simulink model "JUB27_MA"  (R2020b)
settings: Solver=FixedStepDiscrete  StartTime=0.0  StopTime=2*3600  FixedStep=Ts  RelTol=1e-3
values from neighbouring files (symbols this model uses):
  FreqAlvoIni = 55    [CarregaDados.m]
  NumCasasDecimais = 1    [CarregaDados.m]
  PMonAlvoIni = LimitaFaixa(PMonAlvoIni,FaixaPChegada)    [CarregaDados.m]
  Rede_Processo = load('weightsESNx_TR300_TVaz0.8_RaioE0.1.mat')    [CarregaDados.m]
  SNR = 40    [CarregaDados.m]
  Ts = 10    [CarregaDados.m]
undefined symbols (not defined in the file or in its folder): awgn, BTP, TabelaIsometricas, TabSimulador, UIni, YIni
settings Model: Creator=leize  LastModifiedBy=leize

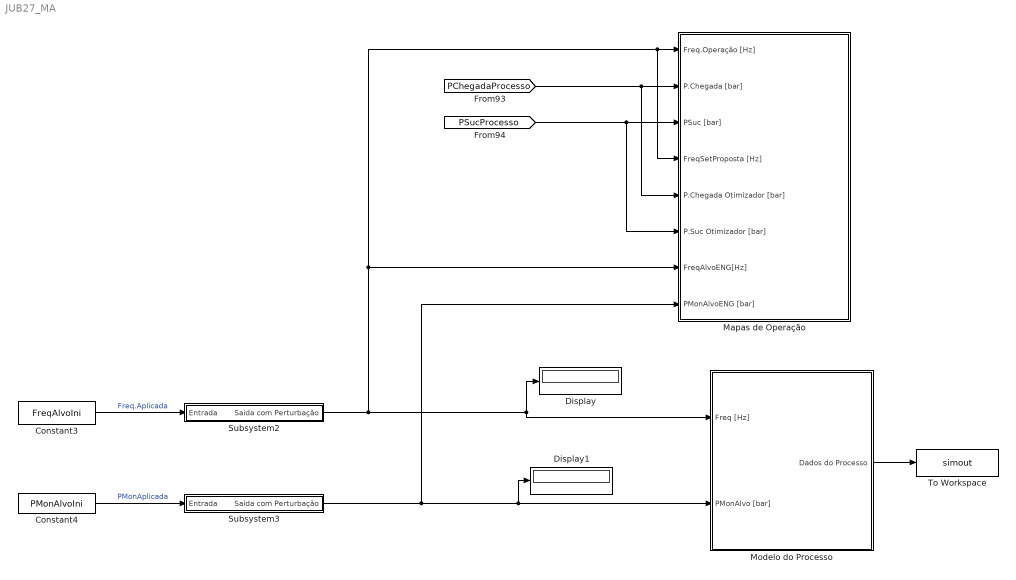
== system JUB27_MA ==
  Constant3 : Constant  Value=FreqAlvoIni
  Constant4 : Constant  Value=PMonAlvoIni
  Display : Display
  Display1 : Display
  Mapas de Operação : Subsystem  mask{PlotaMapas=1, HabilitaRastro=1, Tsim=TabSimulador, BTP=BTP, TabelaIsometricas=TabelaIsometricas, FreqIni=UIni(1), PChegadaIni=YIni(2), PSucIni=YIni(1), FreqAlvoIni=FreqAlvoIni, PMonAlvoIni=PMonAlvoIni}
      mask prompts: PlotaMapas "Plotar Mapas (1/0)?"; HabilitaRastro "Habilita Rastro do Plot (1/0)?"; Tsim "Tabela do Simulador"; BTP "Tabela BTP"; TabelaIsometricas "Tabela Curvas Isometricas"; FreqIni "Frequencia Inicial [Hz]"; PChegadaIni "PChegada Inicial [bar]"; PSucIni "Pressao de Succao Inicial [bar]"; FreqAlvoIni "Frequencia ALVO Inicial [Hz]"; PMonAlvoIni "PChegada ALVO [bar]"
      mask DialogControl DescTextVar Prompt: MAPAS DE OPERAÇÃO
      mask DialogControl ParameterGroupVar Prompt: Tabelas Petrobras e configurações dos Mapas de Operação
      mask DialogControl ParameterGroupVar_copy Prompt: Dados do Processo
      mask DialogControl ParameterGroupVar_copy_copy_copy Prompt: Dados Engenharia (Alvos)
  Modelo do Processo : Subsystem  mask{ESN=Rede_Processo, YIni=YIni, UIni=UIni, SNR=SNR, NumCasasDecimais=NumCasasDecimais}
      mask prompts: ESN "Estruturada ESN"; YIni "Condicoes iniciais das variaveis"; UIni "Condicao Inicial das manipuladas (Freq e PMon)"; SNR "Relação Sinal Ruido aplicada"; NumCasasDecimais "Numero de casas decimais"
  Subsystem2 : Subsystem  mask{TIni=1*3600, DeltaT=3600, ValorP=0}
      mask prompts: TIni "Tempo Inicio"; DeltaT "Duracao"; ValorP "Valor da Perturbacao"
  Subsystem3 : Subsystem  mask{TIni=3*3600, DeltaT=3600, ValorP=0}
      mask prompts: TIni "Tempo Inicio"; DeltaT "Duracao"; ValorP "Valor da Perturbacao"
  To Workspace : ToWorkspace  VariableName=simout  SaveFormat=Timeseries  SampleTime=-1
  wires:
  Modelo do Processo/1(Dados do Processo) -> To Workspace/1
  [PSucProcesso] -> Mapas de Operação/6(P.Suc Otimizador [bar]), Mapas de Operação/3(PSuc [bar])
  [PChegadaProcesso] -> Mapas de Operação/2(P.Chegada [bar]), Mapas de Operação/5(P.Chegada Otimizador [bar])
  Constant4/1 -> Subsystem3/1(Entrada)  "PMonAplicada"
  Constant3/1 -> Subsystem2/1(Entrada)  "Freq.Aplicada"
  Subsystem3/1(Saida com Perturbação) -> Mapas de Operação/8(PMonAlvoENG [bar]), Display1/1, Modelo do Processo/2(PMonAlvo [bar])
  Subsystem2/1(Saida com Perturbação) -> Mapas de Operação/7(FreqAlvoENG[Hz]), Mapas de Operação/4(FreqSetProposta [Hz]), Mapas de Operação/1(Freq.Operação [Hz]), Modelo do Processo/1(Freq [Hz]), Display/1

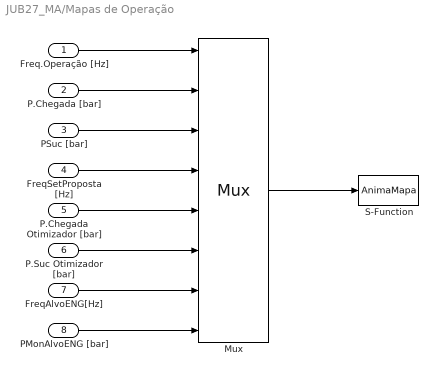
== system JUB27_MA/Mapas de Operação ==
  Freq.Operação [Hz] : Inport
  P.Chegada [bar] : Inport  Port=2
  PSuc [bar] : Inport  Port=3
  FreqSetProposta [Hz] : Inport  Port=4
  P.Chegada Otimizador [bar] : Inport  Port=5
  P.Suc Otimizador [bar] : Inport  Port=6
  FreqAlvoENG[Hz] : Inport  Port=7
  PMonAlvoENG [bar] : Inport  Port=8
  Mux : Mux  Inputs=8
  S-Function : S-Function  FunctionName=AnimaMapa  Parameters=PlotaMapas,Tsim,BTP,FreqIni, PChegadaIni,PSucIni,FreqAlvoIni,PMonAlvoIni,HabilitaRastro,TabelaIsometricas  SFunctionDeploymentMode=off  EnableBusSupport=off
  wires:
  Freq.Operação [Hz]/1 -> Mux/1
  Mux/1 -> S-Function/1
  P.Chegada [bar]/1 -> Mux/2
  PSuc [bar]/1 -> Mux/3
  P.Chegada Otimizador [bar]/1 -> Mux/5
  P.Suc Otimizador [bar]/1 -> Mux/6
  FreqAlvoENG[Hz]/1 -> Mux/7
  PMonAlvoENG [bar]/1 -> Mux/8
  FreqSetProposta [Hz]/1 -> Mux/4

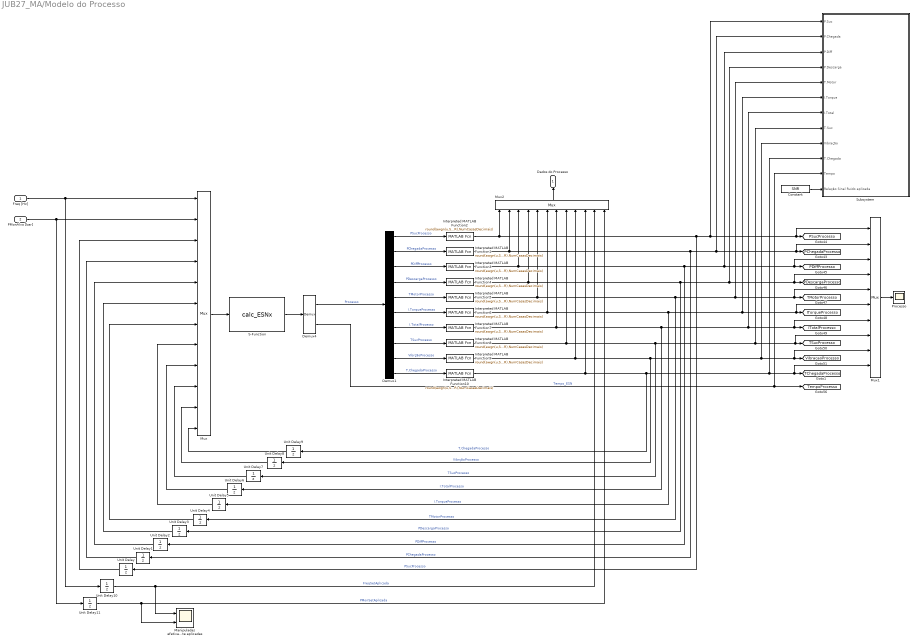
== system JUB27_MA/Modelo do Processo ==
  Freq [Hz] : Inport
  PMonAlvo [bar] : Inport  Port=2
  Constant : Constant  Value=SNR
  Demux1 : Demux  Outputs=10
  Demux4 : Demux  Outputs="[ 10  1]"
  Interpreted MATLAB Function{1..10} (10 alike) : MATLABFcn  MATLABFcn=round(awgn(u,SNR),NumCasasDecimais)
  Manipuladas efetivamente aplicadas : Scope  NumInputPorts=2
  Mux : Mux  Inputs=2+10
  Mux1 : Mux  Inputs=10
  Mux2 : Mux  Inputs=12
  Processo : Scope
  S-Function : S-Function  FunctionName=calc_ESNx  Parameters=ESN.data,YIni  SFunctionDeploymentMode=off  EnableBusSupport=off
  Subsystem : Subsystem
  Unit Delay : UnitDelay  InitialCondition=YIni(1)  SampleTime=-1  HasFrameUpgradeWarning=on
  Unit Delay1 : UnitDelay  InitialCondition=YIni(2)  SampleTime=-1  HasFrameUpgradeWarning=on
  Unit Delay10 : UnitDelay  InitialCondition=UIni(1)  SampleTime=-1  HasFrameUpgradeWarning=on
  Unit Delay11 : UnitDelay  InitialCondition=UIni(2)  SampleTime=-1  HasFrameUpgradeWarning=on
  Unit Delay2 : UnitDelay  InitialCondition=YIni(3)  SampleTime=-1  HasFrameUpgradeWarning=on
  Unit Delay3 : UnitDelay  InitialCondition=YIni(4)  SampleTime=-1  HasFrameUpgradeWarning=on
  Unit Delay4 : UnitDelay  InitialCondition=YIni(5)  SampleTime=-1  HasFrameUpgradeWarning=on
  Unit Delay5 : UnitDelay  InitialCondition=YIni(6)  SampleTime=-1  HasFrameUpgradeWarning=on
  Unit Delay6 : UnitDelay  InitialCondition=YIni(7)  SampleTime=-1  HasFrameUpgradeWarning=on
  Unit Delay7 : UnitDelay  InitialCondition=YIni(8)  SampleTime=-1  HasFrameUpgradeWarning=on
  Unit Delay8 : UnitDelay  InitialCondition=YIni(9)  SampleTime=-1  HasFrameUpgradeWarning=on
  Unit Delay9 : UnitDelay  InitialCondition=YIni(10)  SampleTime=-1  HasFrameUpgradeWarning=on
  Dados do Processo : Outport
  tag scope: ITorqueProcesso=global, ITotalProcesso=global, PChegadaProcesso=global, PDescargaProcesso=global, PDiffProcesso=global, PSucProcesso=global, TChegadaProcesso=global, TMotorProcesso=global, TSucProcesso=global, TempoProcesso=global, VibracaoProcesso=global
  wires:
  Mux/1 -> S-Function/1
  PMonAlvo [bar]/1 -> Unit Delay11/1, Mux/2
  Freq [Hz]/1 -> Mux/1, Unit Delay10/1
  Unit Delay/1 -> Mux/3
  Unit Delay1/1 -> Mux/4
  Unit Delay2/1 -> Mux/5
  Unit Delay3/1 -> Mux/6
  Unit Delay4/1 -> Mux/7
  Unit Delay5/1 -> Mux/8
  Unit Delay6/1 -> Mux/9
  Unit Delay7/1 -> Mux/10
  Unit Delay8/1 -> Mux/11
  Unit Delay9/1 -> Mux/12
  S-Function/1 -> Demux4/1
  Demux1/4 -> Interpreted MATLAB Function4/1  "PDescargaProcesso"
  Demux1/3 -> Interpreted MATLAB Function3/1  "PDiffProcesso"
  Demux1/9 -> Interpreted MATLAB Function9/1  "VibrçãoProcesso"
  Demux1/7 -> Interpreted MATLAB Function7/1  "I.TotalProcesso"
  Demux1/10 -> Interpreted MATLAB Function10/1  "T,ChegadaProcesso"
  Demux4/2 -> Subsystem/11(Tempo), [TempoProcesso]  "Tempo_ESN"
  Mux1/1 -> Processo/1
  Interpreted MATLAB Function2/1 -> Unit Delay/1, Subsystem/1(P.Suc), Mux1/1, [PSucProcesso], Mux2/1  "PSucProcesso"
  Interpreted MATLAB Function1/1 -> Subsystem/2(P.Chegada), Mux1/2, [PChegadaProcesso], Unit Delay1/1, Mux2/2  "PChegadaProcesso"
  Interpreted MATLAB Function3/1 -> Subsystem/3(P.Diff), Mux1/3, [PDiffProcesso], Unit Delay2/1, Mux2/3  "PDiffProcesso"
  Interpreted MATLAB Function4/1 -> Subsystem/4(P.Descarga), Mux1/4, [PDescargaProcesso], Unit Delay3/1, Mux2/4  "PDescargaProcesso"
  Interpreted MATLAB Function5/1 -> Subsystem/5(T.Motor), Mux1/5, [TMotorProcesso], Unit Delay4/1, Mux2/5  "TMotorProcesso"
  Interpreted MATLAB Function6/1 -> Subsystem/6(I.Torque), Mux1/6, [ITorqueProcesso], Unit Delay5/1, Mux2/6  "I.TorqueProcesso"
  Interpreted MATLAB Function7/1 -> Subsystem/7(I.Total), Mux1/7, [ITotalProcesso], Unit Delay6/1, Mux2/7  "I.TotalProcesso"
  Interpreted MATLAB Function8/1 -> Subsystem/8(T.Suc), Mux1/8, [TSucProcesso], Unit Delay7/1, Mux2/8  "TSucProcesso"
  Interpreted MATLAB Function9/1 -> Subsystem/9(Vibração), Mux1/9, [VibracaoProcesso], Unit Delay8/1, Mux2/9  "VibrçãoProcesso"
  Interpreted MATLAB Function10/1 -> Unit Delay9/1, Mux1/10, [TChegadaProcesso], Subsystem/10(T.Chegada), Mux2/10  "T,ChegadaProcesso"
  Constant/1 -> Subsystem/12(Relação Sinal Ruido aplicada)
  Demux1/1 -> Interpreted MATLAB Function2/1  "PSucProcesso"
  Demux1/2 -> Interpreted MATLAB Function1/1  "PChegadaProcesso"
  Demux1/5 -> Interpreted MATLAB Function5/1  "TMotorProcesso"
  Demux1/6 -> Interpreted MATLAB Function6/1  "I.TorqueProcesso"
  Demux1/8 -> Interpreted MATLAB Function8/1  "TSucProcesso"
  Mux2/1 -> Dados do Processo/1
  Demux4/1 -> Demux1/1  "Processo"
  Unit Delay10/1 -> Manipuladas efetivamente aplicadas/1, Mux2/11  "FreqSetAplicada"
  Unit Delay11/1 -> Manipuladas efetivamente aplicadas/2, Mux2/12  "PMonSetAplicada"

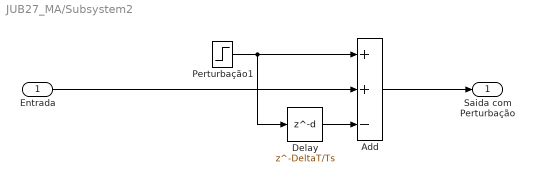
== system JUB27_MA/Subsystem2 ==
  Entrada : Inport
  Add : Sum  Inputs=++-
  Delay : Delay  DelayLength=DeltaT/Ts
  Perturbação1 : Step  Time=TIni  After=ValorP  SampleTime=0
  Saida com Perturbação : Outport
  wires:
  Perturbação1/1 -> Delay/1, Add/1
  Add/1 -> Saida com Perturbação/1
  Delay/1 -> Add/3
  Entrada/1 -> Add/2

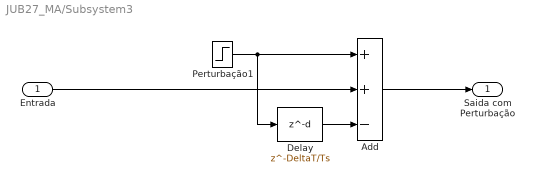
== system JUB27_MA/Subsystem3 ==
  Entrada : Inport
  Add : Sum  Inputs=++-
  Delay : Delay  DelayLength=DeltaT/Ts
  Perturbação1 : Step  Time=TIni  After=ValorP  SampleTime=0
  Saida com Perturbação : Outport
  wires:
  Entrada/1 -> Add/2
  Delay/1 -> Add/3
  Add/1 -> Saida com Perturbação/1
  Perturbação1/1 -> Add/1, Delay/1

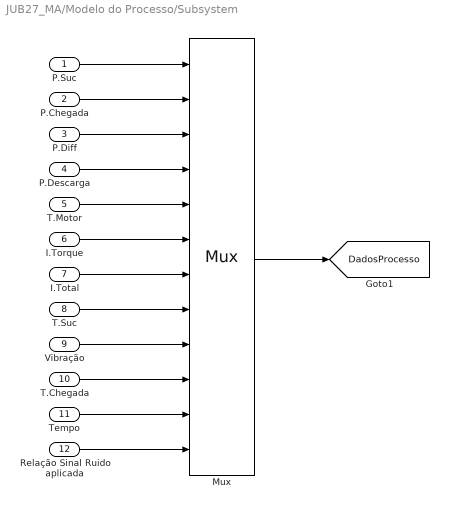
== system JUB27_MA/Modelo do Processo/Subsystem ==
  P.Suc : Inport
  P.Chegada : Inport  Port=2
  P.Diff : Inport  Port=3
  P.Descarga : Inport  Port=4
  T.Motor : Inport  Port=5
  I.Torque : Inport  Port=6
  I.Total : Inport  Port=7
  T.Suc : Inport  Port=8
  Vibração : Inport  Port=9
  T.Chegada : Inport  Port=10
  Tempo : Inport  Port=11
  Relação Sinal Ruido aplicada : Inport  Port=12
  Mux : Mux  Inputs=12
  tag scope: DadosProcesso=global
  wires:
  P.Suc/1 -> Mux/1
  P.Chegada/1 -> Mux/2
  T.Motor/1 -> Mux/5
  I.Torque/1 -> Mux/6
  T.Suc/1 -> Mux/8
  P.Diff/1 -> Mux/3
  I.Total/1 -> Mux/7
  P.Descarga/1 -> Mux/4
  Mux/1 -> [DadosProcesso]
  T.Chegada/1 -> Mux/10
  Vibração/1 -> Mux/9
  Tempo/1 -> Mux/11
  Relação Sinal Ruido aplicada/1 -> Mux/12
